simulink model "joystick_example"  (R2018b)
settings: Solver=VariableStepAuto  StartTime=0.0  StopTime=30.0  RelTol=1e-3
libraries: joystick_lib x1, aerolibanimutils x1
settings Model: Creator=Yannic  LastModifiedBy=yannic
settings DataIOCC: SaveOutput=off  SaveTime=off

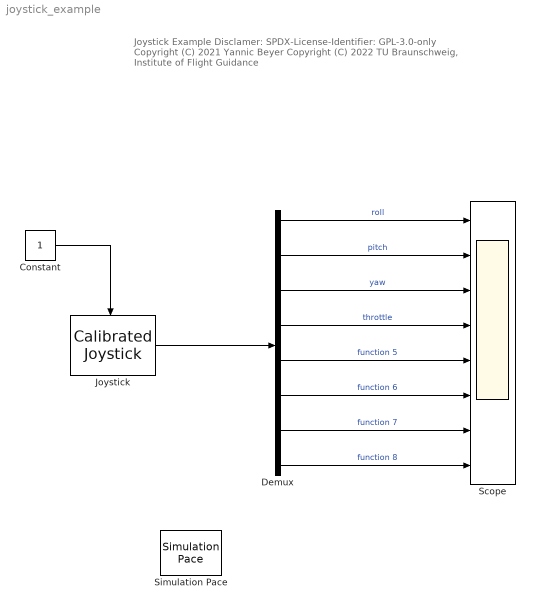
== system joystick_example ==
  note: Joystick Example
      |
      | Disclamer:
      | SPDX-License-Identifier: GPL-3.0-only
      |
      | Copyright (C) 2021 Yannic Beyer
      | Copyright (C) 2022 TU Braunschweig, Institute of Flight Guidance
  Constant : Constant
  Demux : Demux  Outputs=8
  Joystick : joystick_lib/Calibrated Joystick  jystck=jystck
      settings: SourceProductName=LADAC
  Scope : Scope  NumInputPorts=8
  Simulation Pace : aerolibanimutils/Simulation Pace  SimulationPace=1  SleepMode=Auto  OutputPaceError=off  SampleTime=1/30
  wires:
  Joystick/1 -> Demux/1
  Demux/1 -> Scope/1  "roll"
  Demux/2 -> Scope/2  "pitch"
  Demux/3 -> Scope/3  "yaw"
  Demux/4 -> Scope/4  "throttle"
  Demux/5 -> Scope/5  "function 5"
  Demux/6 -> Scope/6  "function 6"
  Demux/7 -> Scope/7  "function 7"
  Demux/8 -> Scope/8  "function 8"
  Constant/1 -> Joystick/Enable
